simulink model "martins_version_wconv_wdc_wWT"  (R2023b)
settings: Solver=VariableStepAuto  StartTime=0.0  StopTime=30  RelTol=1.0e-3
undefined symbols (not defined in the file): C_dc, c_drt, c_f, C_hv_km, C_p_opt, Cagg, DiscIntNeverNeededParam, G_dc_denom, G_dc_num, H_gen, H_vsm, H_WTR, Ibase_hv, Ibase_lv, Ibase_mv, k_AD, k_d_vsm, k_decouple, k_drt, k_ffv, k_ic, k_idc, k_mod, k_p_p_vsm, k_p_q_vsm, k_pc, k_pdc, K_pitch, ki_dc, KI_LL, ki_q, kp_dc, KP_LL, kslope_VSC, L_comp, L_d, l_f, l_f_si1, l_grid, L_hv_km, L_q, l_t_ehvhv, l_t_hvmv, l_t_mvlv, L_Virt, Lagg, lambda_opt, Lbase1v, length_export, omega_nom, omega_WTR_min, omega_WTR_n, omega_WTR_sl, P_aero_0, phase_shift_test_state, phase_shifts, pie_export, pitch_max, pitch_min, Pitchanglevector ... (+40)
libraries: slpidlib x9, spsFirstOrderFilterLib x3, simulink x1, spsSampleandHoldLib x1, spspowerguiLib x1
(part 1 of 4)
settings Model: SimulationMode=accelerator  Creator=marti  LastModifiedBy=Martin Pedersen
settings DataIOCC: MaxDataPoints=590000  SaveOperatingPoint=on  SaveFormat=Array  SaveOutput=off  SaveTime=off

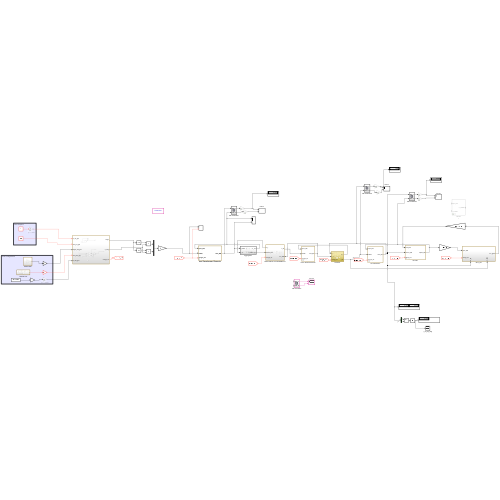
[thumbnail: Simulink's stored preview of the top-level diagram]
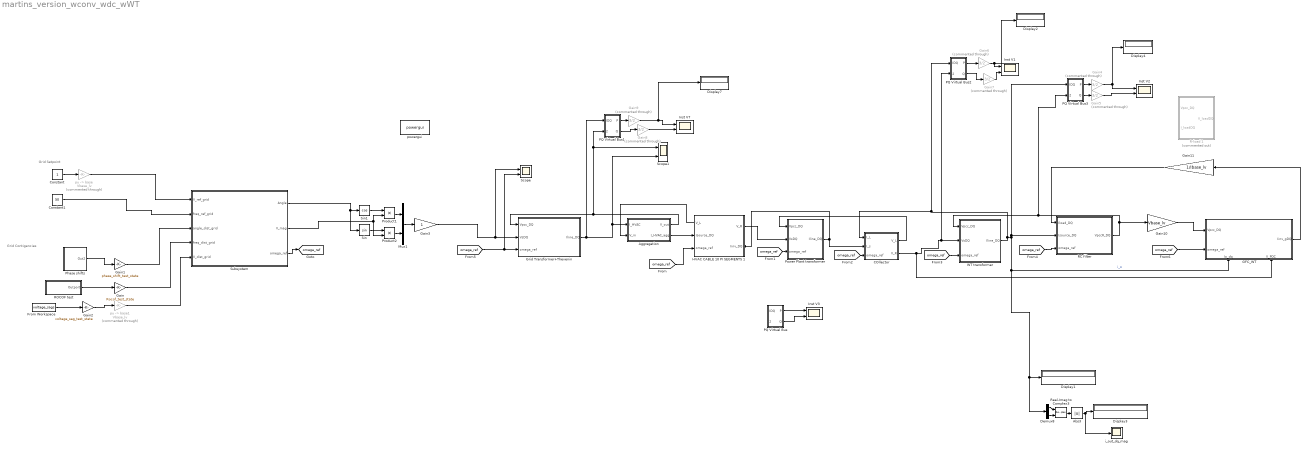
== system martins_version_wconv_wdc_wWT ==
  note: Grid Contigencies
  note: Grid Setpoint
  Abs3 : Abs
  Aggregation : Subsystem
  COllector : Subsystem
  Constant : Constant  SampleTime=Ts_power
  Constant1 : Constant  Value=50  SampleTime=Ts_power
  Demux8 : Demux  Outputs=[vect vect]
  Display{1..4,7} (5 alike) : Display
  From Workspace : FromWorkspace  VariableName=voltage_sags
  GFC_WT : Subsystem
      settings: PortSchema="{\"entries\":[{\"content\":{\"sides\":[{\"content\":{\"connectorIds\":[\"In1\",\"In2\"]},\"type\":\"ConnectorPlacement.EquallySpacedRectSide\",\"uuid\":\"b1342998-2362-446f-8f57-ef2b1b89f54b\"},{\"content\":{\"connectorIds\":[\"Out1\"],\"side\":\"RIGHT\"},\"type\":\"ConnectorPlacement.EquallySpacedRectSide\",\"uuid\":\"a510629f-f2f1-4b6f-afed-16515a5df6be\"},{\"content\":{\"side\":\"TOP\"},\"type\":\"ConnectorPlacement.EquallySpacedRectSide\",\"uuid\":\"1296e810-4d4d-483a-bdac-d12a6e4c4bea\"},{\"content\":{\"connectorIds\":[\"In3\",\"In4\"],\"side\":\"BOTTOM\"},\"type\":\"ConnectorPlacement.EquallySpacedRectSide\",\"uuid\":\"e381b032-cba3-4396-8af6-dd7d6efe00c5\"}]},\"type\":\"ConnectorPlacement.EquallySpacedConnector\",\"uuid\":\"9087b561-963f-43c4-b5d6-329d0df97dbb\"}],\"packageUris\":[\"http://schema.mathworks.com/mf0/Connector/R2020b\"],\"version\":\"1.0\"}"
  Gain : Gain  Gain=Rocof_test_state
  Gain1 : Gain  Gain=phase_shift_test_state
  Gain10 : Gain  Gain=Vbase_lv
  Gain11 : Gain  Gain=1/Ibase_lv
  Gain2 : Gain  Gain=voltage_sag_test_state
  Gain3 : Gain  SaturateOnIntegerOverflow=on  OutDataTypeStr=Inherit: Same as input  ParamDataTypeStr=Inherit: Same as input
  Gain{4..9} (6 alike) : Gain  Commented=through  Gain=3/2
  Grid Transformer+Thevenin : Subsystem  mask{Rsource=r_grid+r_t_ehvhv, Lsource=(l_grid+l_t_ehvhv)/omega_nom}
      mask prompts: Rsource "Line resistance"; Lsource "line inductance"
      mask help:
      | RLV_NET is an 3 phase series RL with no virtual resistance termination,
      | 2 voltages as inputs and 1 current output
      mask init:
      | inv_Lsource=1/Lsource;
      mask TypeOptions Rsource: 2/Gain | 3/Gain
      mask TypeOptions Lsource: 7/Gain
  HVAC CABLE 10 PI SEGMENTS 1 : Subsystem
      settings: PortSchema="{\"entries\":[{\"content\":{\"sides\":[{\"content\":{\"connectorIds\":[\"Out2\",\"In1\",\"In2\"]},\"type\":\"ConnectorPlacement.EquallySpacedRectSide\",\"uuid\":\"364e0a5e-18fb-4479-9cea-0c32c2a31756\"},{\"content\":{\"connectorIds\":[\"Out1\",\"In3\"],\"side\":\"RIGHT\"},\"type\":\"ConnectorPlacement.EquallySpacedRectSide\",\"uuid\":\"1b6ff004-fcad-4add-afdc-525ba11bb75d\"},{\"content\":{\"side\":\"TOP\"},\"type\":\"ConnectorPlacement.EquallySpacedRectSide\",\"uuid\":\"fcc13093-d95c-447e-b2c0-1261755b0002\"}]},\"type\":\"ConnectorPlacement.EquallySpacedConnector\",\"uuid\":\"424862c2-d061-479a-b3c0-8c92e3670b7a\"}],\"packageUris\":[\"http://schema.mathworks.com/mf0/Connector/R2020b\"],\"version\":\"1.0\"}"
  Inst V{1..3,7} (4 alike) : Scope  NumInputPorts=2
  Mux1 : Mux  Inputs=2
  PQ Virtual Bus : Subsystem
  PQ Virtual Bus1 : Subsystem
  PQ Virtual Bus2 : Subsystem
  PQ Virtual Bus3 : Subsystem
  Phase shifts : Subsystem
  Power Plant transformer : Subsystem  mask{Rsource=r_t_hvmv, Lsource=l_t_hvmv/omega_nom}
      mask prompts: Rsource "Line resistance"; Lsource "line inductance"
      mask help:
      | RLV_NET is an 3 phase series RL with no virtual resistance termination,
      | 2 voltages as inputs and 1 current output
      mask init:
      | inv_Lsource=1/Lsource;
      mask TypeOptions Rsource: 2/Gain | 3/Gain
      mask TypeOptions Lsource: 7/Gain
  Product1 : Product
  Product2 : Product
  R-load 1 : Subsystem  Commented=on  mask{Rsource=1, Lsource=0}
      mask prompts: Rsource "Line resistance"; Lsource "line inductance"
      mask help:
      | RLV_NET is an 3 phase series RL with no virtual resistance termination,
      | 2 voltages as inputs and 1 current output
      mask init:
      | inv_Lsource=1/Lsource;
      mask TypeOptions Rsource: 2/Gain | 3/Gain
      mask TypeOptions Lsource: 7/Gain
  RC filter : Subsystem  mask{Csource=c_f/omega_nom, Rd=0, VD0=1, VQ0=0}
      mask prompts: Csource "Net Capacitance"; Rd "Rdamp"
      mask help:
      | PI network, capacitance to enter is total.
      | Left and right current as input. Left and right voltage as output
      mask init:
      | inv_Csource=1/Csource;
      mask TypeOptions Csource: 8/Gain
      mask TypeOptions Rd: 1/Gain | 2/Gain
      mask TypeOptions VD0: VcpdR_int/InitialCondition
      mask TypeOptions VQ0: VcpqR_int/InitialCondition
  ROCOF test : Subsystem
  Real-Imag to Complex3 : RealImagToComplex
  Scope : Scope  NumInputPorts=2
  Scope1 : Scope  NumInputPorts=2
  Sin : Trigonometry
  Sin1 : Trigonometry  Operator=cos
  Subsystem : Subsystem
  "WT transformer " : Subsystem  mask{Rsource=r_t_mvlv, Lsource=l_t_mvlv/omega_nom}
      mask prompts: Rsource "Line resistance"; Lsource "line inductance"
      mask help:
      | RLV_NET is an 3 phase series RL with no virtual resistance termination,
      | 2 voltages as inputs and 1 current output
      mask init:
      | inv_Lsource=1/Lsource;
      mask TypeOptions Rsource: 2/Gain | 3/Gain
      mask TypeOptions Lsource: 7/Gain
  i_out_dq_mag : Scope
  powergui : spspowerguiLib/powergui  Priority=1  SimulationMode=Continuous  SampleTime=Ts_power  frequency=60  Iterations=50  frequencyindice=60  Pbase=100e6  ErrMax=1e-4  UnitsV=kV  UnitsW=MW  buscounter=0  FunctionMessages=off  echomessages=off  EnableUseOfTLC=off  CurrentSourceSwitches=off  DisableSnubberDevices=off  DisableRonSwitches=off  DisableVfSwitches=off  DisplayEquations=off  AutomaticDiscreteSolvers=off  SolverType=Tustin/Backward Euler (TBE)  Interpol=off  ExternalGateDelay=off  methode=off  Ts=100  x0status=blocks  SPID=on  SwTol=0  HookPort=off  NonlinearTolerance=1e-4  nMaxIteration=100  ContinueOnMaxIteration=off  RestoreLinks=warning  ResistiveCurrentMeasurement=off  Frange=[0:2:500]  Ylog=off  Xlog=on  ShowGrid=off  save=off  variable=ZData  structure=0  ZoomFFT=off  StartTime=0.0  cycles=1  DisplayStyle=1  fundamental=60  FreqAxis=off  MaxFrequency=1000  frequencyindicesteady=1  RmsSteady=1  display=off
  "pu -> base" : Gain  Commented=through  Gain=Vbase_lv
  "pu -> base1" : Gain  Commented=through  Gain=Vbase_lv
  tag scope: omega_ref=global
  wires:
  "pu -> base"/1 -> Subsystem/1(V_ref_grid)
  ROCOF test/1(Outport) -> Gain/1
  "pu -> base1"/1 -> Subsystem/5(V_dist_grid)
  Constant1/1 -> Subsystem/2(freq_ref_grid)
  Gain2/1 -> "pu -> base1"/1
  Phase shifts/1(Out2) -> Gain1/1
  Gain/1 -> Subsystem/4(freq_dist_grid)
  Gain1/1 -> Subsystem/3(angle_dist_grid)
  Constant/1 -> "pu -> base"/1
  From Workspace/1 -> Gain2/1
  Mux1/1 -> Gain3/1
  Sin/1 -> Product2/1
  Sin1/1 -> Product1/1
  Product2/1 -> Mux1/2
  Subsystem/1(Angle) -> Sin/1, Sin1/1
  Product1/1 -> Mux1/1
  Subsystem/2(V_mag) -> Product2/2, Product1/2
  Gain3/1 -> Scope/1, Grid Transformer+Thevenin/2("VsDQ ")
  Subsystem/3(omega_ref) -> [omega_ref]
  [omega_ref] -> Scope/2, Grid Transformer+Thevenin/3(omega_ref)
  Grid Transformer+Thevenin/1(Iline_DQ) -> Aggregation/1(I_HVAC), Scope1/2, PQ Virtual Bus1/1(IDQ)
  [omega_ref] -> HVAC CABLE 10 PI SEGMENTS 1/2(omega_ref)
  [omega_ref] -> Power Plant transformer/3(omega_ref)
  [omega_ref] -> COllector/3(omega_ref)
  [omega_ref] -> RC filter/3(omega_ref)
  Aggregation/1(V_out) -> PQ Virtual Bus1/2(VDQ), Scope1/1, Grid Transformer+Thevenin/1(Vpcc_DQ)
  PQ Virtual Bus/1(P) -> Inst V3/1
  PQ Virtual Bus/2(Q) -> Inst V3/2
  PQ Virtual Bus1/1(P) -> Gain9/1
  PQ Virtual Bus1/2(Q) -> Gain8/1
  Real-Imag to Complex3/1 -> Abs3/1
  "WT transformer "/1(Iline_DQ) -> PQ Virtual Bus2/1(IDQ), COllector/1(I_L), Demux8/1, Display1/1, GFC_WT/3(Io_dq), RC filter/2("Isource_DQ "), PQ Virtual Bus3/1(IDQ)  "i_o"
  Abs3/1 -> i_out_dq_mag/1, Display3/1
  Demux8/2 -> Real-Imag to Complex3/2
  Demux8/1 -> Real-Imag to Complex3/1
  Gain11/1 -> RC filter/1(Iload_DQ)
  [omega_ref] -> "WT transformer "/3(omega_ref)
  [omega_ref] -> GFC_WT/2(omega_ref)
  Gain10/1 -> GFC_WT/1(Vpcc_DQ)
  GFC_WT/1(Iinv_gDQ) -> Gain11/1
  PQ Virtual Bus2/2(Q) -> Gain7/1
  PQ Virtual Bus2/1(P) -> Gain6/1
  COllector/2(V_R) -> PQ Virtual Bus2/2(VDQ), "WT transformer "/2("VsDQ "), GFC_WT/4(V_POC)
  PQ Virtual Bus3/1(P) -> Gain4/1
  PQ Virtual Bus3/2(Q) -> Gain5/1
  RC filter/1(VpccR_DQ) -> Gain10/1, "WT transformer "/1(Vpcc_DQ), PQ Virtual Bus3/2(VDQ)
  HVAC CABLE 10 PI SEGMENTS 1/1(V_R) -> Power Plant transformer/2("VsDQ ")
  Aggregation/2(I_HVAC_agg) -> HVAC CABLE 10 PI SEGMENTS 1/1("Isource_DQ ")
  HVAC CABLE 10 PI SEGMENTS 1/2(V_L) -> Aggregation/2(V_in)
  Power Plant transformer/1(Iline_DQ) -> COllector/2(I_s), HVAC CABLE 10 PI SEGMENTS 1/3(Iinv_DQ)
  COllector/1(V_L) -> Power Plant transformer/1(Vpcc_DQ)
  Gain4/1 -> Display4/1, Inst V2/1
  Gain5/1 -> Inst V2/2
  Gain6/1 -> Inst V1/1, Display2/1
  Gain7/1 -> Inst V1/2
  Gain8/1 -> Inst V7/2
  Gain9/1 -> Display7/1, Inst V7/1

== system martins_version_wconv_wdc_wWT/Aggregation ==
  I_HVAC : Inport
  V_in : Inport  Port=2
  Demux1 : Demux  Outputs=[vect vect]
  Demux2 : Demux  Outputs=2
  Gain2 : Gain  Gain=1/(1*vect)
  Gain3 : Gain  Gain=ones(vect,1)
  Gain4 : Gain  Gain=ones(vect,1)
  Mux2 : Mux  Inputs=2
  Mux3 : Mux  Inputs=2
  Sum of Elements : Sum  Inputs=+
  Sum of Elements1 : Sum  Inputs=+
  V_out : Outport
  I_HVAC_agg : Outport  Port=2
  wires:
  Mux3/1 -> Gain2/1
  Gain3/1 -> Mux2/1
  Demux2/1 -> Gain3/1
  Sum of Elements1/1 -> Mux3/2
  Gain4/1 -> Mux2/2
  Demux2/2 -> Gain4/1
  Sum of Elements/1 -> Mux3/1
  Gain2/1 -> I_HVAC_agg/1
  V_in/1 -> Demux2/1
  Mux2/1 -> V_out/1
  I_HVAC/1 -> Demux1/1
  Demux1/1 -> Sum of Elements/1
  Demux1/2 -> Sum of Elements1/1

== system martins_version_wconv_wdc_wWT/COllector ==
  I_L : Inport
  I_s : Inport  Port=2
  omega_ref : Inport  Port=3
  Gain2 : Gain  Gain=1/Vbase_mv
  Gain3 : Gain  Gain=1/Vbase_mv
  Gain4 : Gain  Gain=Ibase_mv
  Gain5 : Gain  Gain=Ibase_mv
  Scope : Scope  NumInputPorts=2
  collector : Subsystem  mask{Rsource=Ragg, Csource=Cagg, Lsource=Lagg}
      mask prompts: Rsource "Series R"; Csource "Net Capacitance"; Lsource "Net Inductance"
      mask help:
      | PI network, capacitance to enter is total.
      | Left and right current as input. Left and right voltage as output
      mask init:
      | inv_Csource=2/Csource;
      | inv_Lsource=1/Lsource;
      mask TypeOptions Rsource: 2/Gain | 3/Gain
      mask TypeOptions Csource: 8/Gain
      mask TypeOptions Lsource: 7/Gain
  V_L : Outport
  V_R : Outport  Port=2
  wires:
  Gain4/1 -> collector/1(Iload_DQ)
  collector/1(VpccR_DQ) -> Gain2/1
  Gain2/1 -> V_R/1
  collector/2(VpccL_DQ) -> Gain3/1
  I_s/1 -> Gain5/1
  Gain3/1 -> Scope/1, V_L/1
  Gain5/1 -> collector/2("Isource_DQ ")
  I_L/1 -> Scope/2, Gain4/1
  omega_ref/1 -> collector/3(omega_ref)

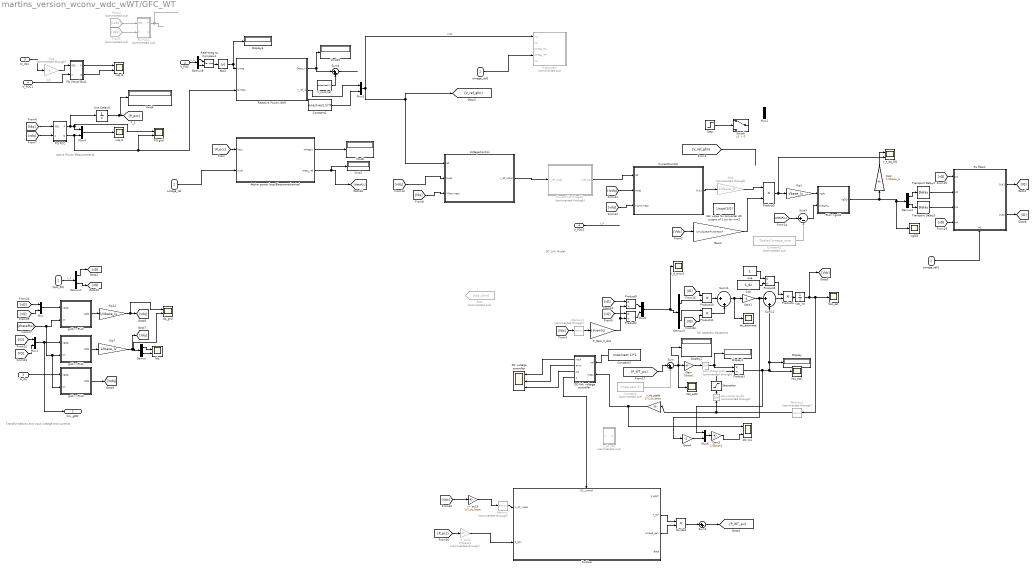
== system martins_version_wconv_wdc_wWT/GFC_WT ==
  note: DC Link Model
  note: Active Power Measurements
  note: Transformations and input voltage and currents
  note: DC capacitor equations
  Vpcc_DQ : Inport
  omega_ref : Inport  Port=2
  Io_dq : Inport  Port=3
  V_POC : Inport  Port=4
  -> pu12 : Gain  Commented=through  Gain=1/Sbase1
  -> pu13 : Gain  Gain=1/V_dc_base
  Abs3 : Abs
  Active power loop/Electromechanical : Subsystem
  "Cdc " : Constant  Value=C_dc
  Constant : Constant  Commented=on  Value=ones(vect,1)
  Constant1 : Constant  Value=ones(vect,1)*0
  Constant2 : Constant  Commented=on  Value=Tdelay*omega_nom
  Constant7 : Constant  Value=ones(vect,1)*1
  Current Limit Logic1 : Subsystem  Commented=through
  CurrentControl : Subsystem
  DC link : Scope  NumInputPorts=2
  DC voltage controller : Scope  NumInputPorts=3
  DC-link voltage controller : Subsystem
  Demux : Demux  Outputs=2
  Demux1 : Demux  Outputs=[vect vect]
  Demux2 : Demux  Outputs=2
  Demux3 : Demux  Outputs=2
  Demux8 : Demux  Outputs=[vect vect]
  Display{,1..2,4} (4 alike) : Display
  Divide1 : Product  Inputs=**
  From4 : From  Commented=on  GotoTag=Iodq
  From5 : From  Commented=on  GotoTag=vdq
  Gain : Gain  Gain=Sbase1
  Gain1 : Gain  Gain=-1
  Gain2 : Gain  Gain=1/(V_dc_base)*1/(sqrt(3/2))
  Gain3 : Gain  Gain=1/Sbase1
  Gain4 : Gain  Gain=-1
  Goto : Goto  Commented=on  GotoTag=Idq_ulim
  I_d_error1 : Scope
  Idc_estimate : Scope
  Idq : Scope  NumInputPorts=2
  Io_dq1 : InportShadow  Port=3
  Kip1 : Gain  Gain=Vbase_lv
  Kip14 : Gain  Gain=1/Vbase_lv
  Kip2 : Gain  Gain=1/Vbase_lv
  Kip3 : Gain  Commented=through  Gain=1/Vbase_lv
  Kip4 : Gain  Commented=through  Gain=-1
  Kip7 : Gain  Gain=1/Ibase_lv
  Memory : Memory  Commented=through  InitialCondition=1
  Memory1 : Memory  Commented=through  InitialCondition=V_dc
  Memory2 : Memory  Commented=through  InitialCondition=V_dc
  Mux{,2..6} (6 alike) : Mux  Inputs=2
  Mux1 : Mux  Inputs=[vect vect]
  PLL>>grid1 : Subsystem  AncestorBlock=powerlib_meascontrol/Transformations/Alpha-Beta-Zero to dq0/Subsystem - pi//2 delay
  PQ PCC : Subsystem
  PQ PCC1 : Subsystem  Commented=on
  PQ Virtual Bus1 : Subsystem
  PQ grid : Scope  NumInputPorts=2
  P_Gain_V_dc2 : Gain  Gain=0.5*sqrt(3/2)
  Product{1..3,9} (4 alike) : Product  Inputs=*/
  Product10 : Product  Inputs=**
  Product11 : Product  Inputs=**
  Product4 : Product  Inputs=**
  Product5 : Product  Inputs=**  InputSameDT=on  SaturateOnIntegerOverflow=on  OutDataTypeStr=Inherit: Same as first input
  RL filter1 : Subsystem
      settings: PortSchema="{\"entries\":[{\"content\":{\"sides\":[{\"content\":{\"connectorIds\":[\"In1\",\"In2\",\"In3\",\"In4\"]},\"type\":\"ConnectorPlacement.EquallySpacedRectSide\",\"uuid\":\"57ad71d1-5664-4b35-a20c-d71f7e1cdc47\"},{\"content\":{\"connectorIds\":[\"Out1\",\"Out2\"],\"side\":\"RIGHT\"},\"type\":\"ConnectorPlacement.EquallySpacedRectSide\",\"uuid\":\"8101605d-eedb-4c26-847d-0cc0ce629d60\"},{\"content\":{\"connectorIds\":[],\"side\":\"TOP\"},\"type\":\"ConnectorPlacement.EquallySpacedRectSide\",\"uuid\":\"2627b00b-24a5-469a-be2d-9c3c8a1d2080\"},{\"content\":{\"connectorIds\":[\"In5\"],\"side\":\"BOTTOM\"},\"type\":\"ConnectorPlacement.EquallySpacedRectSide\",\"uuid\":\"fe553db7-7727-4a02-b1e7-5aedfb7840ee\"}]},\"type\":\"ConnectorPlacement.EquallySpacedConnector\",\"uuid\":\"f40200c8-ad5b-428c-8a4e-7641595b86c4\"}],\"packageUris\":[\"http://schema.mathworks.com/mf0/Connector/19700101\"],\"version\":\"1.0\"}"
  Reactive Power /AVR : Subsystem
  Real-Imag to Complex3 : RealImagToComplex
  Saturation : Saturate  UpperLimit=10000  LowerLimit=100
  Step : Step  Before=1  After=0  SampleTime=0
  Subsystem : Subsystem  Commented=on
  Sum{,2,4,11..12} (5 alike) : Sum  Inputs=|++
  Sum5 : Sum  Inputs=|+-
  Switch : Switch  Criteria=u2 > Threshold  SaturateOnIntegerOverflow=off  InputSameDT=off
  Transport Delay2 : TransportDelay  DelayTime=Tdelay/4  BufferSize=3560000
  Transport Delay3 : TransportDelay  DelayTime=Tdelay/4  BufferSize=3560000
  Turbine : Subsystem
      settings: PortSchema="{\"entries\":[{\"content\":{\"sides\":[{\"content\":{\"connectorIds\":[\"In1\",\"In2\"]},\"type\":\"ConnectorPlacement.EquallySpacedRectSide\",\"uuid\":\"21e34078-e55f-4d30-b877-fe893009bf50\"},{\"content\":{\"connectorIds\":[\"Out1\",\"Out2\",\"Out3\",\"Out4\"],\"side\":\"RIGHT\"},\"type\":\"ConnectorPlacement.EquallySpacedRectSide\",\"uuid\":\"7fcce3d7-4700-4aed-9466-c9df21636c23\"},{\"content\":{\"side\":\"TOP\"},\"type\":\"ConnectorPlacement.EquallySpacedRectSide\",\"uuid\":\"1e7dcbfc-6914-4635-b5b6-37bd72b5c977\"},{\"content\":{\"connectorIds\":[\"In3\"],\"side\":\"BOTTOM\"},\"type\":\"ConnectorPlacement.EquallySpacedRectSide\",\"uuid\":\"4cd2ac35-fe5e-4d2f-8870-f4b31c475178\"}]},\"type\":\"ConnectorPlacement.EquallySpacedConnector\",\"uuid\":\"0de0e372-1be9-4afb-8b34-f97f900b0306\"}],\"packageUris\":[\"http://schema.mathworks.com/mf0/Connector/R2020b\"],\"version\":\"1.0\"}"
  Unit Delay9 : UnitDelay  SampleTime=Ts_power  StateName='p_pcc'  HasFrameUpgradeWarning=on
  V_POC1 : InportShadow  Port=4
  V_POC2 : InportShadow  Port=4
  V_nominal : Constant  Value=ones(vect,1)
  Vdc value for converter AC output of 1 pu for m=2 : Constant  Value=1/sqrt(3/2)
  Vdc_est : Scope
  Vdc_est1 : Scope
  Vdc_est2 : Scope
  "Vdc_int " : Integrator  Priority=1  InitialCondition=V_dc  UpperSaturationLimit=300  LowerSaturationLimit=-100  ContinuousStateAttributes='v_dc'
  Vmd{1,4,8,15} (4 alike) : Display
  VoltageControl : Subsystem
  Zero-Order Hold1 : ZeroOrderHold  Commented=through  SampleTime=Ts_power
  Zero-Order Hold2 : ZeroOrderHold  Commented=through  SampleTime=Ts_power
  dq_grid : Scope  NumInputPorts=2
  grid>>PLL1 : Subsystem  AncestorBlock=powerlib_meascontrol/Transformations/dq0 to Alpha-Beta-Zero/Subsystem1
  grid>>PLL2 : Subsystem  AncestorBlock=powerlib_meascontrol/Transformations/dq0 to Alpha-Beta-Zero/Subsystem1
  grid>>PLL3 : Subsystem  AncestorBlock=powerlib_meascontrol/Transformations/dq0 to Alpha-Beta-Zero/Subsystem1
  omega_ref1 : InportShadow  Port=2
  omega_ref2 : InportShadow  Port=2
  one : Constant
  v_dc_reg : Subsystem  Commented=on
  "v_dc_scale " : Gain  Gain=1/V_dc_base  SaturateOnIntegerOverflow=on  OutDataTypeStr=Inherit: Same as input  ParamDataTypeStr=Inherit: Same as input
  v_t_dq_DQ : Scope  NumInputPorts=2
  vdq 6 : Scope
  vdq 8 : Scope  NumInputPorts=2
  vgDQ : Scope
  Iinv_gDQ : Outport  VectorParamsAs1DForOutWhenUnconnected=off
  wires:
  Active power loop/Electromechanical/2(Theta_ref) -> [thetaPLL], Vmd1/1
  Active power loop/Electromechanical/1(omega1) -> Vmd8/1
  [P_pcc] -> Active power loop/Electromechanical/1(Ppcc)
  Unit Delay9/1 -> [P_pcc], Vmd4/1
  PQ PCC/1(P) -> Mux4/1, PQ grid/1, Unit Delay9/1
  omega_ref/1 -> Active power loop/Electromechanical/2(wref)
  Constant1/1 -> Mux3/2
  Demux/1 -> Idq/1
  grid>>PLL2/1(vgdq) -> Kip14/1
  Demux/2 -> Idq/2
  Mux1/1 -> grid>>PLL1/1(vgDQ), Iinv_gDQ/1
  grid>>PLL1/1(vgdq) -> Kip7/1
  Mux/1 -> grid>>PLL2/1(vgDQ)
  [IQ] -> Mux1/2
  [thetaPLL] -> grid>>PLL2/2(wt), grid>>PLL1/2(wt), grid>>PLL3/2(wt)
  [ID] -> Mux1/1
  [vD] -> Mux/1
  [vQ] -> Mux/2
  Io_dq/1 -> grid>>PLL3/1(vgDQ)
  grid>>PLL3/1(vgdq) -> [Iodq]
  [vdq] -> PQ PCC/2(VDQ)
  [Idq] -> PQ PCC/1(IDQ)
  Kip7/1 -> dq_grid/2, Demux/1, [Idq]
  Kip14/1 -> dq_grid/1, [vdq]
  PQ PCC/2(Q) -> PQ grid/2, Reactive Power /AVR/2(Qmeas), Mux4/2
  Mux4/1 -> vdq 6/1
  Abs3/1 -> Display4/1, Reactive Power /AVR/1(Vmag)
  Demux8/2 -> Real-Imag to Complex3/2
  Demux8/1 -> Real-Imag to Complex3/1
  Real-Imag to Complex3/1 -> Abs3/1
  Io_dq1/1 -> Kip4/1
  Sum4/1 -> ?
  Reactive Power /AVR/1(Delta_V) -> Vmd15/1, Sum4/1
  V_nominal/1 -> Sum4/2
  PQ Virtual Bus1/1(P) -> vdq 8/1
  Vpcc_DQ/1 -> Demux1/1  "v_o"
  Demux1/2 -> [vQ]
  Demux1/1 -> [vD]
  V_POC1/1 -> PQ Virtual Bus1/2(VDQ)  "v_o"
  V_POC/1 -> Demux8/1  "v_o"
  "v_dc_scale "/1 -> DC link/1, DC-link voltage controller/2(meas)
  Product2/1 -> Mux5/2
  Zero-Order Hold2/1 -> Product1/1, Display1/1
  Demux3/2 -> Product11/1
  P_Gain_V_dc2/1 -> Product9/2, Product2/2
  Gain1/1 -> Gain4/1, Sum12/1
  "Vdc_int "/1 -> [Vdc], Memory1/1, Vdc_est/1
  [vQ] -> Product2/1
  Saturation/1 -> Product1/2
  Sum12/1 -> Product4/2
  Product10/1 -> Sum11/1
  [IQ] -> Product11/2
  DC-link voltage controller/4(DC_control) -> Turbine/3(DC_control)
  Product4/1 -> "Vdc_int "/1
  Product11/1 -> Sum11/2
  [ID] -> Product10/1
  Demux3/1 -> Product10/2
  Sum/1 -> Vdc_est2/1, Display2/1, Gain/1
  "Cdc "/1 -> Product3/2
  Gain/1 -> Zero-Order Hold2/1
  one/1 -> Product3/1
  Sum11/1 -> Gain1/1, Idc_estimate/1
  Product3/1 -> Product4/1
  Product1/1 -> Mux6/1, Display/1, Sum12/2, Vdc_est1/1
  [vD] -> Product9/1
  Constant7/1 -> DC-link voltage controller/1(ref)
  Zero-Order Hold1/1 -> Saturation/1
  Product9/1 -> Mux5/1
  [Vdc] -> Memory2/1
  Mux5/1 -> Demux3/1, I_d_error1/1
  Reactive Power /AVR/2(V_ref_d) -> Mux3/1
  [Idq] -> VoltageControl/3(I filter meas)
  Current Limit Logic1/1(I_ref_sat) -> CurrentControl/1(ref)
  [Iodq] -> CurrentControl/2(meas)
  V_POC2/1 -> ?  "v_o"
  Constant2/1 -> Sum5/2
  [thetaPLL] -> Sum5/1
  Product5/1 -> v_t_dq_DQ/2, Kip1/1
  Kip1/1 -> PLL>>grid1/1(vgdq)
  Sum5/1 -> PLL>>grid1/2(thetaPLL)
  [Vdc] -> Gain2/1
  Transport Delay3/1 -> RL filter1/3(In3)
  PLL>>grid1/1(vgDQ) -> vgDQ/1, Demux2/1, Kip2/1
  [vD] -> RL filter1/4(In4)
  omega_ref1/1 -> RL filter1/5(In5)
  [vQ] -> RL filter1/1(In1)
  Demux2/1 -> Transport Delay2/1
  RL filter1/2(Out2) -> [ID]
  RL filter1/1(Out1) -> [IQ]
  Transport Delay2/1 -> RL filter1/2(In2)
  Demux2/2 -> Transport Delay3/1
  [vdq] -> VoltageControl/2(meas)
  omega_ref2/1 -> Subsystem/4(omega_ref)
  Kip3/1 -> Product5/1
  Mux3/1 -> Subsystem/1(In1), VoltageControl/1(ref), [V_ref_gfm]  "Vref"
  [V_ref_gfm] -> ?
  Step/1 -> Switch/2
  VoltageControl/1(I_ref_unsat) -> Current Limit Logic1/1(I_ref_unsat)
  CurrentControl/1(Out1) -> Kip3/1
  DC-link voltage controller/3(out) -> DC voltage controller/3
  DC-link voltage controller/2(error) -> DC voltage controller/2
  DC-link voltage controller/1(input) -> DC voltage controller/1
  Gain2/1 -> Product5/2
  PQ PCC1/1(P) -> ?
  From4/1 -> PQ PCC1/1(IDQ)
  PQ Virtual Bus1/2(Q) -> vdq 8/2
  From5/1 -> PQ PCC1/2(VDQ)
  Memory1/1 -> Zero-Order Hold1/1, "v_dc_scale "/1
  Memory2/1 -> P_Gain_V_dc2/1
  Kip4/1 -> PQ Virtual Bus1/1(IDQ)
  Constant/1 -> Sum/2
  Kip2/1 -> v_t_dq_DQ/1
  Mux6/1 -> Gain3/1
  Gain3/1 -> DC link/2
  Gain4/1 -> Mux6/2
  [vdq] -> CurrentControl/3(V grid meas)
  [P_WT_pu] -> Sum/1
  [Vdc] -> -> pu13/1
  Memory/1 -> Turbine/2(V_dc_meas)
  Turbine/2(omega_gen) -> Divide1/2
  -> pu13/1 -> Memory/1
  Divide1/1 -> Sum2/1
  -> pu12/1 -> Turbine/1(P_gfm)
  Turbine/3(T_em) -> Divide1/1
  [P_pcc] -> -> pu12/1
  Sum2/1 -> [P_WT_pu]

== system martins_version_wconv_wdc_wWT/Grid Transformer+Thevenin ==
  note: Network
  note: VIRTUAL RESITANCE
  Vpcc_DQ : Inport
  "VsDQ " : Inport  Port=2
  omega_ref : Inport  Port=3
  1 : Gain  Gain=inv_Lsource
  2 : Gain  Gain=Rsource
  3 : Gain  Gain=Rsource
  4 : Gain  Gain=inv_Lsource
  7 : Gain  Gain=Lsource
  Demux1 : Demux  Outputs=2
  Demux2 : Demux  Outputs=2
  Id : Scope
  Iline_D_int : Integrator  UpperSaturationLimit=50  LowerSaturationLimit=-1000
  Iline_Q_int : Integrator  UpperSaturationLimit=50  LowerSaturationLimit=-1000
  Iq : Scope
  Mux1 : Mux  Inputs=2
  Mux4 : Mux  Inputs=2
  Product1 : Product
  Product2 : Product
  Sum1 : Sum  Inputs=|+---
  Sum8 : Sum  Inputs=|+-+-
  Iline_DQ : Outport  VectorParamsAs1DForOutWhenUnconnected=off
  wires:
  7/1 -> [wL]
  omega_ref/1 -> 7/1
  [Vpcc_Q] -> Sum1/1
  [Vpcc_D] -> Sum8/1
  Demux2/1 -> Mux4/1, [Vpcc_D]
  Demux2/2 -> Mux4/2, [Vpcc_Q]
  Sum1/1 -> 4/1
  1/1 -> Iline_D_int/1
  Iline_D_int/1 -> Product1/2, Id/1, 2/1, Mux1/1
  Iline_Q_int/1 -> Mux1/2, Iq/1, Product2/2, 3/1
  Sum8/1 -> 1/1
  2/1 -> Sum8/4
  Product2/1 -> Sum8/3
  3/1 -> Sum1/4
  4/1 -> Iline_Q_int/1
  Product1/1 -> Sum1/3
  [wL] -> Product1/1, Product2/1
  Demux1/1 -> Sum8/2
  Demux1/2 -> Sum1/2
  "VsDQ "/1 -> Demux1/1
  Vpcc_DQ/1 -> Demux2/1
  Mux1/1 -> Iline_DQ/1

== system martins_version_wconv_wdc_wWT/HVAC CABLE 10 PI SEGMENTS 1 ==
  "Isource_DQ " : Inport
  omega_ref : Inport  Port=2
  Iinv_DQ : Inport  Port=3
  Gain1 : Gain  Gain=1/Vbase_hv
  Gain2 : Gain  Gain=1/Vbase_hv
  Gain4 : Gain  Gain=Ibase_hv
  Gain5 : Gain  Gain=Ibase_hv
  RC sys1 : Subsystem  mask{Csource=C_hv_km*length_export/pie_export/2, Rd=0.00001, VD0=1, VQ0=0}
      mask prompts: Csource "Net Capacitance"; Rd "Rdamp"
      mask help:
      | PI network, capacitance to enter is total.
      | Left and right current as input. Left and right voltage as output
      mask init:
      | inv_Csource=1/Csource;
      mask TypeOptions Csource: 8/Gain
      mask TypeOptions Rd: 1/Gain | 2/Gain
      mask TypeOptions VD0: VcpdR_int/InitialCondition
      mask TypeOptions VQ0: VcpqR_int/InitialCondition
  RLC_NET 11 : Subsystem  mask{Csource=C_hv_km*length_export/pie_export, Rsource=R_hv_km*length_export/pie_export, Lsource=L_hv_km*length_export/pie_export}
      mask prompts: Csource "line capacitance 1 side"; Rsource "Line resistance"; Lsource "line inductance"
      mask help:
      | RL with C terminations on right,
      | Left Voltage  and Right current input, Right voltage and left current output
      mask init:
      | inv_Csource=1/Csource;
      | inv_Lsource=1/Lsource;
      mask TypeOptions Csource: 8/Gain
      mask TypeOptions Rsource: 2/Gain | 3/Gain
      mask TypeOptions Lsource: 7/Gain
  RLC_NET 12 : Subsystem  mask{Csource=C_hv_km*length_export/pie_export, Rsource=R_hv_km*length_export/pie_export, Lsource=L_hv_km*length_export/pie_export}
      mask prompts: Csource "line capacitance 1 side"; Rsource "Line resistance"; Lsource "line inductance"
      mask help:
      | RL with C terminations on right,
      | Left Voltage  and Right current input, Right voltage and left current output
      mask init:
      | inv_Csource=1/Csource;
      | inv_Lsource=1/Lsource;
      mask TypeOptions Csource: 8/Gain
      mask TypeOptions Rsource: 2/Gain | 3/Gain
      mask TypeOptions Lsource: 7/Gain
  RLC_NET 13 : Subsystem  mask{Csource=C_hv_km*length_export/pie_export, Rsource=R_hv_km*length_export/pie_export, Lsource=L_hv_km*length_export/pie_export}
      mask prompts: Csource "line capacitance 1 side"; Rsource "Line resistance"; Lsource "line inductance"
      mask help:
      | RL with C terminations on right,
      | Left Voltage  and Right current input, Right voltage and left current output
      mask init:
      | inv_Csource=1/Csource;
      | inv_Lsource=1/Lsource;
      mask TypeOptions Csource: 8/Gain
      mask TypeOptions Rsource: 2/Gain | 3/Gain
      mask TypeOptions Lsource: 7/Gain
  RLC_NET 14 : Subsystem  mask{Csource=C_hv_km*length_export/pie_export, Rsource=R_hv_km*length_export/pie_export, Lsource=L_hv_km*length_export/pie_export}
      mask prompts: Csource "line capacitance 1 side"; Rsource "Line resistance"; Lsource "line inductance"
      mask help:
      | RL with C terminations on right,
      | Left Voltage  and Right current input, Right voltage and left current output
      mask init:
      | inv_Csource=1/Csource;
      | inv_Lsource=1/Lsource;
      mask TypeOptions Csource: 8/Gain
      mask TypeOptions Rsource: 2/Gain | 3/Gain
      mask TypeOptions Lsource: 7/Gain
  RLC_NET 15 : Subsystem  mask{Csource=C_hv_km*length_export/pie_export, Rsource=R_hv_km*length_export/pie_export, Lsource=L_hv_km*length_export/pie_export}
      mask prompts: Csource "line capacitance 1 side"; Rsource "Line resistance"; Lsource "line inductance"
      mask help:
      | RL with C terminations on right,
      | Left Voltage  and Right current input, Right voltage and left current output
      mask init:
      | inv_Csource=1/Csource;
      | inv_Lsource=1/Lsource;
      mask TypeOptions Csource: 8/Gain
      mask TypeOptions Rsource: 2/Gain | 3/Gain
      mask TypeOptions Lsource: 7/Gain
  RLC_NET 16 : Subsystem  mask{Csource=C_hv_km*length_export/pie_export, Rsource=R_hv_km*length_export/pie_export, Lsource=L_hv_km*length_export/pie_export}
      mask prompts: Csource "line capacitance 1 side"; Rsource "Line resistance"; Lsource "line inductance"
      mask help:
      | RL with C terminations on right,
      | Left Voltage  and Right current input, Right voltage and left current output
      mask init:
      | inv_Csource=1/Csource;
      | inv_Lsource=1/Lsource;
      mask TypeOptions Csource: 8/Gain
      mask TypeOptions Rsource: 2/Gain | 3/Gain
      mask TypeOptions Lsource: 7/Gain
  RLC_NET 17 : Subsystem  mask{Csource=C_hv_km*length_export/pie_export, Rsource=R_hv_km*length_export/pie_export, Lsource=L_hv_km*length_export/pie_export}
      mask prompts: Csource "line capacitance 1 side"; Rsource "Line resistance"; Lsource "line inductance"
      mask help:
      | RL with C terminations on right,
      | Left Voltage  and Right current input, Right voltage and left current output
      mask init:
      | inv_Csource=1/Csource;
      | inv_Lsource=1/Lsource;
      mask TypeOptions Csource: 8/Gain
      mask TypeOptions Rsource: 2/Gain | 3/Gain
      mask TypeOptions Lsource: 7/Gain
  RLC_NET 18 : Subsystem  mask{Csource=C_hv_km*length_export/pie_export, Rsource=R_hv_km*length_export/pie_export, Lsource=L_hv_km*length_export/pie_export}
      mask prompts: Csource "line capacitance 1 side"; Rsource "Line resistance"; Lsource "line inductance"
      mask help:
      | RL with C terminations on right,
      | Left Voltage  and Right current input, Right voltage and left current output
      mask init:
      | inv_Csource=1/Csource;
      | inv_Lsource=1/Lsource;
      mask TypeOptions Csource: 8/Gain
      mask TypeOptions Rsource: 2/Gain | 3/Gain
      mask TypeOptions Lsource: 7/Gain
  RLC_NET 19 : Subsystem  mask{Csource=C_hv_km*length_export/pie_export, Rsource=R_hv_km*length_export/pie_export, Lsource=L_hv_km*length_export/pie_export}
      mask prompts: Csource "line capacitance 1 side"; Rsource "Line resistance"; Lsource "line inductance"
      mask help:
      | RL with C terminations on right,
      | Left Voltage  and Right current input, Right voltage and left current output
      mask init:
      | inv_Csource=1/Csource;
      | inv_Lsource=1/Lsource;
      mask TypeOptions Csource: 8/Gain
      mask TypeOptions Rsource: 2/Gain | 3/Gain
      mask TypeOptions Lsource: 7/Gain
  RLC_NET 20 : Subsystem  mask{Csource=C_hv_km*length_export/pie_export/2, Rsource=R_hv_km*length_export/pie_export, Lsource=L_hv_km*length_export/pie_export}
      mask prompts: Csource "line capacitance 1 side"; Rsource "Line resistance"; Lsource "line inductance"
      mask help:
      | RL with C terminations on right,
      | Left Voltage  and Right current input, Right voltage and left current output
      mask init:
      | inv_Csource=1/Csource;
      | inv_Lsource=1/Lsource;
      mask TypeOptions Csource: 8/Gain
      mask TypeOptions Rsource: 2/Gain | 3/Gain
      mask TypeOptions Lsource: 7/Gain
  RLV_NET 1 : Subsystem  mask{Rsource=0, Lsource=L_comp}
      mask prompts: Rsource "Line resistance"; Lsource "line inductance"
      mask help:
      | RLV_NET is an 3 phase series RL with no virtual resistance termination,
      | 2 voltages as inputs and 1 current output
      mask init:
      | inv_Lsource=1/Lsource;
      mask TypeOptions Rsource: 2/Gain | 3/Gain
      mask TypeOptions Lsource: 7/Gain
  RLV_NET 2 : Subsystem  mask{Rsource=0, Lsource=L_comp}
      mask prompts: Rsource "Line resistance"; Lsource "line inductance"
      mask help:
      | RLV_NET is an 3 phase series RL with no virtual resistance termination,
      | 2 voltages as inputs and 1 current output
      mask init:
      | inv_Lsource=1/Lsource;
      mask TypeOptions Rsource: 2/Gain | 3/Gain
      mask TypeOptions Lsource: 7/Gain
  Sum2 : Sum  Inputs=++|
  Sum3 : Sum  Inputs=-+|
  V_R : Outport
  V_L : Outport  Port=2
  wires:
  RC sys1/1(VpccR_DQ) -> Gain1/1, RLV_NET 1/1(Vpcc_DQ), RLC_NET 11/2("VsDQ ")
  Gain1/1 -> V_L/1
  "Isource_DQ "/1 -> Gain4/1
  RLC_NET 11/1(Iline_DQ) -> RC sys1/1(Iload_DQ)
  Sum2/1 -> RC sys1/2("Isource_DQ ")
  Gain4/1 -> Sum2/2
  RLV_NET 1/1(Iline_DQ) -> Sum2/1
  omega_ref/1 -> [omega_ref]
  [omega_ref] -> RLC_NET 11/3(omega_ref)
  [omega_ref] -> RLC_NET 12/3(omega_ref)
  [omega_ref] -> RLC_NET 14/3(omega_ref)
  [omega_ref] -> RLC_NET 13/3(omega_ref)
  [omega_ref] -> RLC_NET 15/3(omega_ref)
  [omega_ref] -> RLC_NET 20/3(omega_ref)
  [omega_ref] -> RLC_NET 18/3(omega_ref)
  [omega_ref] -> RLC_NET 19/3(omega_ref)
  [omega_ref] -> RLC_NET 16/3(omega_ref)
  [omega_ref] -> RLC_NET 17/3(omega_ref)
  Iinv_DQ/1 -> Gain5/1
  Gain2/1 -> V_R/1
  RLC_NET 20/2(Vpcc_DQ) -> RLV_NET 2/1(Vpcc_DQ), Gain2/1
  Gain5/1 -> Sum3/2
  RLV_NET 2/1(Iline_DQ) -> Sum3/1
  [omega_ref] -> RLV_NET 2/2(omega_ref)
  RLC_NET 11/2(Vpcc_DQ) -> RLC_NET 12/2("VsDQ ")
  RLC_NET 12/1(Iline_DQ) -> RLC_NET 11/1(Iinv_DQ)
  RLC_NET 13/1(Iline_DQ) -> RLC_NET 12/1(Iinv_DQ)
  RLC_NET 12/2(Vpcc_DQ) -> RLC_NET 13/2("VsDQ ")
  RLC_NET 13/2(Vpcc_DQ) -> RLC_NET 14/2("VsDQ ")
  RLC_NET 14/1(Iline_DQ) -> RLC_NET 13/1(Iinv_DQ)
  RLC_NET 14/2(Vpcc_DQ) -> RLC_NET 15/2("VsDQ ")
  RLC_NET 15/1(Iline_DQ) -> RLC_NET 14/1(Iinv_DQ)
  RLC_NET 16/1(Iline_DQ) -> RLC_NET 15/1(Iinv_DQ)
  RLC_NET 17/1(Iline_DQ) -> RLC_NET 16/1(Iinv_DQ)
  RLC_NET 18/1(Iline_DQ) -> RLC_NET 17/1(Iinv_DQ)
  RLC_NET 16/2(Vpcc_DQ) -> RLC_NET 17/2("VsDQ ")
  RLC_NET 15/2(Vpcc_DQ) -> RLC_NET 16/2("VsDQ ")
  RLC_NET 19/1(Iline_DQ) -> RLC_NET 18/1(Iinv_DQ)
  RLC_NET 18/2(Vpcc_DQ) -> RLC_NET 19/2("VsDQ ")
  RLC_NET 17/2(Vpcc_DQ) -> RLC_NET 18/2("VsDQ ")
  RLC_NET 19/2(Vpcc_DQ) -> RLC_NET 20/2("VsDQ ")
  RLC_NET 20/1(Iline_DQ) -> RLC_NET 19/1(Iinv_DQ)
  Sum3/1 -> RLC_NET 20/1(Iinv_DQ)
  [omega_ref] -> RLV_NET 1/2(omega_ref), RC sys1/3(omega_ref)

== system martins_version_wconv_wdc_wWT/PQ Virtual Bus ==
  note: PQ Virtual bus
  IDQ : Inport
  VDQ : Inport  Port=2
  Demux5 : Demux  Outputs=[vect vect]
  Demux6 : Demux  Outputs=[vect vect]
  Product{1,3..5} (4 alike) : Product  InputSameDT=on  SaturateOnIntegerOverflow=on  OutDataTypeStr=Inherit: Same as first input
  Sum : Sum  InputSameDT=on  SaturateOnIntegerOverflow=on  OutDataTypeStr=Inherit: Same as first input
  Sum1 : Sum  Inputs=+-  InputSameDT=on  SaturateOnIntegerOverflow=on  OutDataTypeStr=Inherit: Same as first input
  P : Outport
  Q : Outport  Port=2
  wires:
  Product3/1 -> Sum/1
  Demux5/2 -> Product4/2, Product5/2
  Product4/1 -> Sum/2
  Demux6/1 -> Product5/1, Product3/2
  Demux5/1 -> Product3/1, Product1/2
  Demux6/2 -> Product1/1, Product4/1
  Product1/1 -> Sum1/1
  Product5/1 -> Sum1/2
  Sum1/1 -> Q/1
  IDQ/1 -> Demux5/1
  VDQ/1 -> Demux6/1
  Sum/1 -> P/1

== system martins_version_wconv_wdc_wWT/PQ Virtual Bus1 ==
  note: PQ Virtual bus
  IDQ : Inport
  VDQ : Inport  Port=2
  Demux5 : Demux  Outputs=[vect vect]
  Demux6 : Demux  Outputs=[vect vect]
  Product{1,3..5} (4 alike) : Product  InputSameDT=on  SaturateOnIntegerOverflow=on  OutDataTypeStr=Inherit: Same as first input
  Sum : Sum  InputSameDT=on  SaturateOnIntegerOverflow=on  OutDataTypeStr=Inherit: Same as first input
  Sum1 : Sum  Inputs=+-  InputSameDT=on  SaturateOnIntegerOverflow=on  OutDataTypeStr=Inherit: Same as first input
  P : Outport
  Q : Outport  Port=2
  wires:
  Product3/1 -> Sum/1
  Demux5/2 -> Product4/2, Product5/2
  Product4/1 -> Sum/2
  Demux6/1 -> Product5/1, Product3/2
  Demux5/1 -> Product3/1, Product1/2
  Demux6/2 -> Product1/1, Product4/1
  Product1/1 -> Sum1/1
  Product5/1 -> Sum1/2
  Sum1/1 -> Q/1
  IDQ/1 -> Demux5/1
  VDQ/1 -> Demux6/1
  Sum/1 -> P/1

== system martins_version_wconv_wdc_wWT/PQ Virtual Bus2 ==
  note: PQ Virtual bus
  IDQ : Inport
  VDQ : Inport  Port=2
  Demux5 : Demux  Outputs=[vect vect]
  Demux6 : Demux  Outputs=[vect vect]
  Product{1,3..5} (4 alike) : Product  InputSameDT=on  SaturateOnIntegerOverflow=on  OutDataTypeStr=Inherit: Same as first input
  Sum : Sum  InputSameDT=on  SaturateOnIntegerOverflow=on  OutDataTypeStr=Inherit: Same as first input
  Sum1 : Sum  Inputs=+-  InputSameDT=on  SaturateOnIntegerOverflow=on  OutDataTypeStr=Inherit: Same as first input
  P : Outport
  Q : Outport  Port=2
  wires:
  Sum/1 -> P/1
  VDQ/1 -> Demux6/1
  IDQ/1 -> Demux5/1
  Sum1/1 -> Q/1
  Product5/1 -> Sum1/2
  Product1/1 -> Sum1/1
  Demux6/2 -> Product4/1, Product1/1
  Demux5/1 -> Product1/2, Product3/1
  Demux6/1 -> Product3/2, Product5/1
  Product4/1 -> Sum/2
  Demux5/2 -> Product5/2, Product4/2
  Product3/1 -> Sum/1

== system martins_version_wconv_wdc_wWT/PQ Virtual Bus3 ==
  note: PQ Virtual bus
  IDQ : Inport
  VDQ : Inport  Port=2
  Demux5 : Demux  Outputs=[vect vect]
  Demux6 : Demux  Outputs=[vect vect]
  Product{1,3..5} (4 alike) : Product  InputSameDT=on  SaturateOnIntegerOverflow=on  OutDataTypeStr=Inherit: Same as first input
  Sum : Sum  InputSameDT=on  SaturateOnIntegerOverflow=on  OutDataTypeStr=Inherit: Same as first input
  Sum1 : Sum  Inputs=+-  InputSameDT=on  SaturateOnIntegerOverflow=on  OutDataTypeStr=Inherit: Same as first input
  P : Outport
  Q : Outport  Port=2
  wires:
  Product3/1 -> Sum/1
  Demux5/2 -> Product4/2, Product5/2
  Product4/1 -> Sum/2
  Demux6/1 -> Product5/1, Product3/2
  Demux5/1 -> Product3/1, Product1/2
  Demux6/2 -> Product1/1, Product4/1
  Product1/1 -> Sum1/1
  Product5/1 -> Sum1/2
  Sum1/1 -> Q/1
  IDQ/1 -> Demux5/1
  VDQ/1 -> Demux6/1
  Sum/1 -> P/1

== system martins_version_wconv_wdc_wWT/Phase shifts ==
  Constant : Constant  Value=0
  From Workspace : FromWorkspace  Commented=on  VariableName=phase_shifts  OutputAfterFinalValue=Setting to zero
  Gain : Gain  Gain=-1
  Step : Step  Time=phase_shifts(1,1)  After=phase_shifts(1,2)  SampleTime=Ts_power
  Step1 : Step  Time=phase_shifts(2,1)  After=phase_shifts(2,2)  SampleTime=0
  Step2 : Step  Time=phase_shifts(3,1)  After=phase_shifts(3,2)  SampleTime=0
  Sum1 : Sum  Inputs=++++
  Out2 : Outport
  wires:
  Sum1/1 -> Out2/1
  Step/1 -> Sum1/1
  Constant/1 -> Gain/1
  From Workspace/1 -> ?
  Step1/1 -> Sum1/2
  Step2/1 -> Sum1/3
  Gain/1 -> Sum1/4

== system martins_version_wconv_wdc_wWT/Power Plant transformer ==
  note: Network
  note: VIRTUAL RESITANCE
  Vpcc_DQ : Inport
  "VsDQ " : Inport  Port=2
  omega_ref : Inport  Port=3
  1 : Gain  Gain=inv_Lsource
  2 : Gain  Gain=Rsource
  3 : Gain  Gain=Rsource
  4 : Gain  Gain=inv_Lsource
  7 : Gain  Gain=Lsource
  Demux1 : Demux  Outputs=[vect vect]
  Demux2 : Demux  Outputs=[vect vect]
  Id : Scope
  Iline_D_int : Integrator  UpperSaturationLimit=50  LowerSaturationLimit=-1000
  Iline_Q_int : Integrator  UpperSaturationLimit=50  LowerSaturationLimit=-1000
  Iq : Scope
  Mux1 : Mux  Inputs=[vect vect]
  Mux4 : Mux  Inputs=[vect vect]
  Product1 : Product
  Product2 : Product
  Sum1 : Sum  Inputs=|+---
  Sum8 : Sum  Inputs=|+-+-
  Iline_DQ : Outport  VectorParamsAs1DForOutWhenUnconnected=off
  wires:
  7/1 -> [wL]
  [Vpcc_Q] -> Sum1/1
  [Vpcc_D] -> Sum8/1
  Demux2/1 -> Mux4/1, [Vpcc_D]
  Demux2/2 -> Mux4/2, [Vpcc_Q]
  Sum1/1 -> 4/1
  1/1 -> Iline_D_int/1
  Iline_D_int/1 -> Product1/2, Id/1, 2/1, Mux1/1
  Iline_Q_int/1 -> Mux1/2, Iq/1, Product2/2, 3/1
  Sum8/1 -> 1/1
  2/1 -> Sum8/4
  Product2/1 -> Sum8/3
  3/1 -> Sum1/4
  4/1 -> Iline_Q_int/1
  Product1/1 -> Sum1/3
  [wL] -> Product1/1, Product2/1
  Demux1/1 -> Sum8/2
  Demux1/2 -> Sum1/2
  "VsDQ "/1 -> Demux1/1
  Vpcc_DQ/1 -> Demux2/1
  Mux1/1 -> Iline_DQ/1
  omega_ref/1 -> 7/1

== system martins_version_wconv_wdc_wWT/R-load 1 ==
  note: Network
  note: VIRTUAL RESITANCE
  note: Shunt R load
  Vpcc_DQ : Inport
  I_loadDQ : Inport  Port=2
  1 : Gain  Commented=on  Gain=inv_Lsource
  2 : Gain  Commented=on  Gain=Rsource
  3 : Gain  Commented=on  Gain=Rsource
  4 : Gain  Commented=on  Gain=inv_Lsource
  7 : Gain  Commented=on  Gain=Lsource
  Demux1 : Demux  Outputs=2
  Demux2 : Demux  Outputs=2
  From2 : From  Commented=on  GotoTag=Vpcc_D
  From28 : From  Commented=on  GotoTag=wL
  From3 : From  Commented=on  GotoTag=Vpcc_Q
  Gain : Gain  Gain=Rsource
  Gain1 : Gain  Gain=Rsource
  Goto2 : Goto  Commented=on  GotoTag=wL
  Id : Scope  Commented=on
  Iline_D_int : Integrator  Commented=on  UpperSaturationLimit=50  LowerSaturationLimit=-1000
  Iline_Q_int : Integrator  Commented=on  UpperSaturationLimit=50  LowerSaturationLimit=-1000
  Iq : Scope  Commented=on
  Mux1 : Mux  Commented=on  Inputs=2
  Mux2 : Mux  Inputs=2
  Mux4 : Mux  Inputs=2
  Product1 : Product  Commented=on
  Product2 : Product  Commented=on
  Sum1 : Sum  Commented=on  Inputs=|+--
  Sum8 : Sum  Commented=on  Inputs=|++-
  V_loadDQ : Outport  VectorParamsAs1DForOutWhenUnconnected=off
  wires:
  Mux1/1 -> ?
  Product2/1 -> Sum8/2
  3/1 -> Sum1/2
  7/1 -> Goto2/1
  From3/1 -> Sum1/1
  From2/1 -> Sum8/1
  Demux2/1 -> Mux4/1, [Vpcc_D]
  Demux2/2 -> Mux4/2, [Vpcc_Q]
  Sum1/1 -> 4/1
  1/1 -> Iline_D_int/1
  Iline_D_int/1 -> Product1/2, Id/1, 2/1, Mux1/1
  Iline_Q_int/1 -> Mux1/2, Iq/1, Product2/2, 3/1
  Sum8/1 -> 1/1
  2/1 -> Sum8/3
  4/1 -> Iline_Q_int/1
  Product1/1 -> Sum1/3
  From28/1 -> Product1/1, Product2/1
  Vpcc_DQ/1 -> Demux2/1
  ? -> 7/1
  Demux1/1 -> Gain/1
  Gain/1 -> Mux2/1
  Mux2/1 -> V_loadDQ/1
  Demux1/2 -> Gain1/1
  Gain1/1 -> Mux2/2
  I_loadDQ/1 -> Demux1/1

== system martins_version_wconv_wdc_wWT/RC filter ==
  note: shunt capacitor
  note: Left shunt capacitor
  Iload_DQ : Inport
  "Isource_DQ " : Inport  Port=2
  omega_ref : Inport  Port=3
  1 : Gain  Commented=on  Gain=Rd
  10 : Gain  Gain=inv_Csource
  2 : Gain  Commented=on  Gain=Rd
  8 : Gain  Gain=Csource
  9 : Gain  Gain=inv_Csource
  Demux2 : Demux  Outputs=2
  Demux3 : Demux  Outputs=2
  Display1 : Display
  Display6 : Display
  Mux1 : Mux  Inputs=2
  Mux2 : Mux  Inputs=2
  Product7 : Product
  Product8 : Product
  Sum1 : Sum  Inputs=|++
  Sum14 : Sum  Inputs=|+--
  Sum15 : Sum  Inputs=|++-
  Sum2 : Sum  Inputs=|++
  Sum3 : Sum  Inputs=|+-
  Sum4 : Sum  Inputs=|+-
  Vcd : Scope
  VcpdR_int : Integrator  InitialCondition=VD0  UpperSaturationLimit=50  LowerSaturationLimit=-1000
  VcpqR_int : Integrator  InitialCondition=VQ0  UpperSaturationLimit=50  LowerSaturationLimit=-1000
  Vcq : Scope
  VpccR_DQ : Outport  VectorParamsAs1DForOutWhenUnconnected=off
  wires:
  Sum4/1 -> 2/1
  Sum3/1 -> 1/1
  Mux2/1 -> Display6/1
  2/1 -> Sum1/2
  1/1 -> Sum2/2
  Sum2/1 -> Mux1/2
  Sum1/1 -> Mux1/1
  VcpdR_int/1 -> Sum1/1, Product8/2, Vcd/1, Mux2/2
  Demux3/1 -> Sum15/3, Sum4/2
  Demux3/2 -> Sum14/2, Sum3/2
  "Isource_DQ "/1 -> Demux3/1
  Iload_DQ/1 -> Demux2/1
  Demux2/2 -> Sum14/1, Sum3/1
  Demux2/1 -> Sum15/2, Sum4/1
  9/1 -> VcpdR_int/1
  Sum14/1 -> 10/1
  [wcs] -> Product8/1, Product7/1
  VcpqR_int/1 -> Vcq/1, Product7/2, Sum2/1, Mux2/1
  Product7/1 -> Sum15/1
  10/1 -> VcpqR_int/1
  Sum15/1 -> 9/1
  Product8/1 -> Sum14/3
  Mux1/1 -> VpccR_DQ/1
  8/1 -> Display1/1, [wcs]
  omega_ref/1 -> 8/1

== system martins_version_wconv_wdc_wWT/ROCOF test ==
  Clock : Clock
  Constant4 : Constant  Value=0
  Constant5 : Constant
  Ramp : simulink/Sources/Ramp  slope=rocof_slope  start=Trocof_start  InitialOutput=0
  Sample and Hold : spsSampleandHoldLib/Sample and Hold  ic=0  Ts=Ts_power
      settings: LibrarySourceBlock=|
      | sps_lib/Control/Sample and
      | Hold
  Switch : Switch  Criteria=u2 > Threshold  Threshold=Trocof_start  SaturateOnIntegerOverflow=off  InputSameDT=off
  Switch1 : Switch  Threshold=Trocof_end  SaturateOnIntegerOverflow=off  InputSameDT=off
  Outport : Outport
  wires:
  Clock/1 -> Switch/2, Switch1/2
  Constant4/1 -> Switch/3, Switch1/1
  Sample and Hold/1 -> Outport/1
  Ramp/1 -> Switch/1
  Constant5/1 -> Switch1/3
  Switch/1 -> Sample and Hold/1
  Switch1/1 -> Sample and Hold/2

== system martins_version_wconv_wdc_wWT/Subsystem ==
  V_ref_grid : Inport
  freq_ref_grid : Inport  Port=2
  angle_dist_grid : Inport  Port=3
  freq_dist_grid : Inport  Port=4
  V_dist_grid : Inport  Port=5
  Constant1 : Constant  Value=0
  Gain : Gain  Gain=2*pi
  Gain1 : Gain  Gain=1/50
  Gain2 : Gain  Gain=2*pi
  Integrator : Integrator
  Integrator1 : Integrator
  Scope : Scope  NumInputPorts=2
  Step : Step  Time=8  After=-0.1963  SampleTime=0
  Sum : Sum  Inputs=|-++
  Sum1 : Sum  Inputs=|+++
  Sum2 : Sum  Inputs=|++
  Angle : Outport
  V_mag : Outport  Port=2
  omega_ref : Outport  Port=3
  wires:
  Constant1/1 -> Gain1/1
  Gain1/1 -> Sum1/3
  Sum/1 -> Angle/1
  V_ref_grid/1 -> Sum2/1
  Sum1/1 -> Gain/1
  V_dist_grid/1 -> Sum2/2, Scope/1
  Sum2/1 -> V_mag/1, Scope/2
  freq_ref_grid/1 -> Sum1/1
  Gain/1 -> omega_ref/1, Integrator/1
  angle_dist_grid/1 -> Sum/3
  freq_dist_grid/1 -> Gain2/1, Sum1/2
  Gain2/1 -> Integrator1/1
  Integrator1/1 -> ?

== system martins_version_wconv_wdc_wWT/WT transformer  ==
  note: Network
  note: VIRTUAL RESITANCE
  Vpcc_DQ : Inport
  "VsDQ " : Inport  Port=2
  omega_ref : Inport  Port=3
  1 : Gain  Gain=inv_Lsource
  2 : Gain  Gain=Rsource
  3 : Gain  Gain=Rsource
  4 : Gain  Gain=inv_Lsource
  7 : Gain  Gain=Lsource
  Demux1 : Demux  Outputs=2
  Demux2 : Demux  Outputs=2
  Id : Scope
  Iline_D_int : Integrator  UpperSaturationLimit=50  LowerSaturationLimit=-1000
  Iline_Q_int : Integrator  UpperSaturationLimit=50  LowerSaturationLimit=-1000
  Iq : Scope
  Mux1 : Mux  Inputs=2
  Mux4 : Mux  Inputs=2
  Product1 : Product
  Product2 : Product
  Sum1 : Sum  Inputs=|+---
  Sum8 : Sum  Inputs=|+-+-
  Iline_DQ : Outport  VectorParamsAs1DForOutWhenUnconnected=off
  wires:
  7/1 -> [wL]
  [Vpcc_Q] -> Sum1/1
  [Vpcc_D] -> Sum8/1
  Demux2/1 -> Mux4/1, [Vpcc_D]
  Demux2/2 -> Mux4/2, [Vpcc_Q]
  Sum1/1 -> 4/1
  1/1 -> Iline_D_int/1
  Iline_D_int/1 -> Product1/2, Id/1, 2/1, Mux1/1
  Iline_Q_int/1 -> Mux1/2, Iq/1, Product2/2, 3/1
  Sum8/1 -> 1/1
  2/1 -> Sum8/4
  Product2/1 -> Sum8/3
  3/1 -> Sum1/4
  4/1 -> Iline_Q_int/1
  Product1/1 -> Sum1/3
  [wL] -> Product1/1, Product2/1
  Demux1/1 -> Sum8/2
  Demux1/2 -> Sum1/2
  "VsDQ "/1 -> Demux1/1
  Vpcc_DQ/1 -> Demux2/1
  Mux1/1 -> Iline_DQ/1
  omega_ref/1 -> 7/1

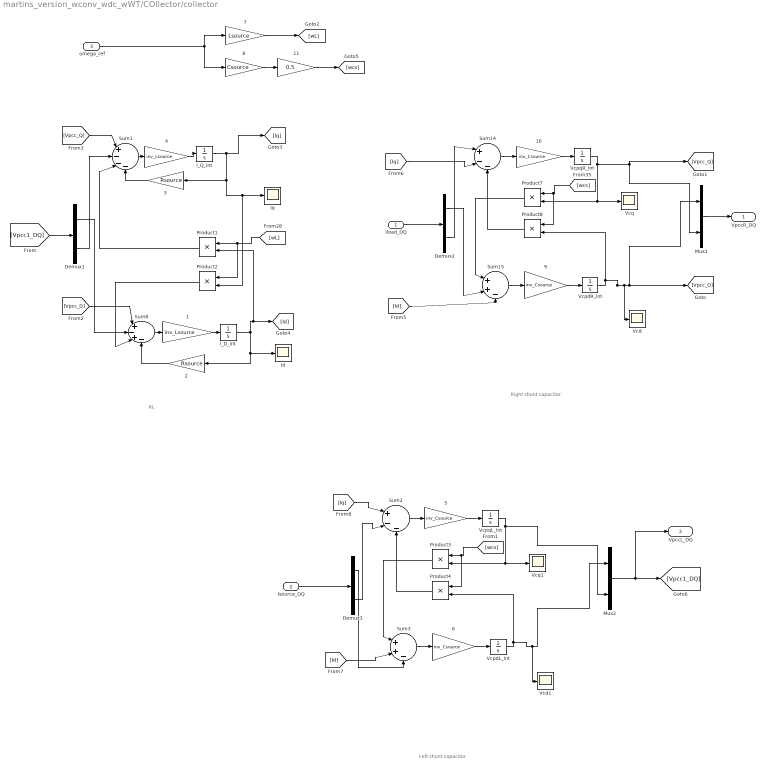
== system martins_version_wconv_wdc_wWT/COllector/collector ==
  note: RL
  note: Right shunt capacitor
  note: Left shunt capacitor
  Iload_DQ : Inport
  "Isource_DQ " : Inport  Port=2
  omega_ref : Inport  Port=3
  1 : Gain  Gain=inv_Lsource
  {5..6,9..10} (4 alike) : Gain  Gain=inv_Csource
  11 : Gain  Gain=0.5
  2 : Gain  Gain=Rsource
  3 : Gain  Gain=Rsource
  4 : Gain  Gain=inv_Lsource
  7 : Gain  Gain=Lsource
  8 : Gain  Gain=Csource
  Demux1 : Demux  Outputs=2
  Demux2 : Demux  Outputs=2
  Demux3 : Demux  Outputs=2
  I_D_int : Integrator  UpperSaturationLimit=50  LowerSaturationLimit=-1000
  I_Q_int : Integrator  UpperSaturationLimit=50  LowerSaturationLimit=-1000
  Id : Scope
  Iq : Scope
  Mux1 : Mux  Inputs=2
  Mux2 : Mux  Inputs=2
  Product{1..4,7..8} (6 alike) : Product
  Sum1 : Sum  Inputs=|+---
  Sum14 : Sum  Inputs=|+--
  Sum15 : Sum  Inputs=|++-
  Sum2 : Sum  Inputs=|+--
  Sum3 : Sum  Inputs=|++-
  Sum8 : Sum  Inputs=|+-+-
  Vcd : Scope
  Vcd1 : Scope
  VcpdL_int : Integrator  UpperSaturationLimit=50  LowerSaturationLimit=-1000
  VcpdR_int : Integrator  UpperSaturationLimit=50  LowerSaturationLimit=-1000
  VcpqL_int : Integrator  UpperSaturationLimit=50  LowerSaturationLimit=-1000
  VcpqR_int : Integrator  UpperSaturationLimit=50  LowerSaturationLimit=-1000
  Vcq : Scope
  Vcq1 : Scope
  VpccR_DQ : Outport  VectorParamsAs1DForOutWhenUnconnected=off
  VpccL_DQ : Outport  Port=2  VectorParamsAs1DForOutWhenUnconnected=off
  wires:
  Iload_DQ/1 -> Demux2/1
  Demux2/2 -> Sum14/1
  Demux2/1 -> Sum15/2
  [wL] -> Product2/1, Product1/1
  Product1/1 -> Sum1/3
  4/1 -> I_Q_int/1
  3/1 -> Sum1/4
  Product2/1 -> Sum8/3
  2/1 -> Sum8/4
  Sum8/1 -> 1/1
  I_Q_int/1 -> 3/1, Product2/2, Iq/1, [Iq]
  I_D_int/1 -> 2/1, Id/1, Product1/2, [Id]
  1/1 -> I_D_int/1
  Sum1/1 -> 4/1
  [Vpcc_D] -> Sum8/1
  [Vpcc_Q] -> Sum1/1
  omega_ref/1 -> 8/1, 7/1
  7/1 -> [wL]
  9/1 -> VcpdR_int/1
  Sum14/1 -> 10/1
  [wcs] -> Product8/1, Product7/1
  [Id] -> Sum15/3
  VcpqR_int/1 -> Mux1/2, [Vpcc_Q], Product7/2, Vcq/1
  Product7/1 -> Sum15/1
  [Iq] -> Sum14/2
  10/1 -> VcpqR_int/1
  Sum15/1 -> 9/1
  Product8/1 -> Sum14/3
  8/1 -> 11/1
  VcpdR_int/1 -> Product8/2, Mux1/1, [Vpcc_D], Vcd/1
  Mux1/1 -> VpccR_DQ/1
  Demux1/1 -> Sum8/2
  Demux1/2 -> Sum1/2
  [Vpcc1_DQ] -> Demux1/1
  VcpdL_int/1 -> Vcd1/1, Mux2/1, Product4/2
  Product4/1 -> Sum2/3
  Sum3/1 -> 6/1
  5/1 -> VcpqL_int/1
  Demux3/2 -> Sum2/2
  Product3/1 -> Sum3/1
  VcpqL_int/1 -> Vcq1/1, Product3/2, Mux2/2
  [wcs] -> Product3/1, Product4/1
  Sum2/1 -> 5/1
  6/1 -> VcpdL_int/1
  "Isource_DQ "/1 -> Demux3/1
  Demux3/1 -> Sum3/3
  [Id] -> Sum3/2
  [Iq] -> Sum2/1
  Mux2/1 -> VpccL_DQ/1, [Vpcc1_DQ]
  11/1 -> [wcs]
